simulink model "problem2"  (R2020a)
settings: Solver=VariableStepAuto  StartTime=0.0  StopTime=100  RelTol=1e-3
model workspace (MAT data in the model file):
  b = 350
  k1 = 80000
  k2 = 500000
  m1 = 2500
  m2 = 320
settings Model: OrderedModelArguments=off  Creator=Jake  LastModifiedBy=Jake
settings DataIOCC: ExternalInput=[t,input ]  LoadExternalInput=on

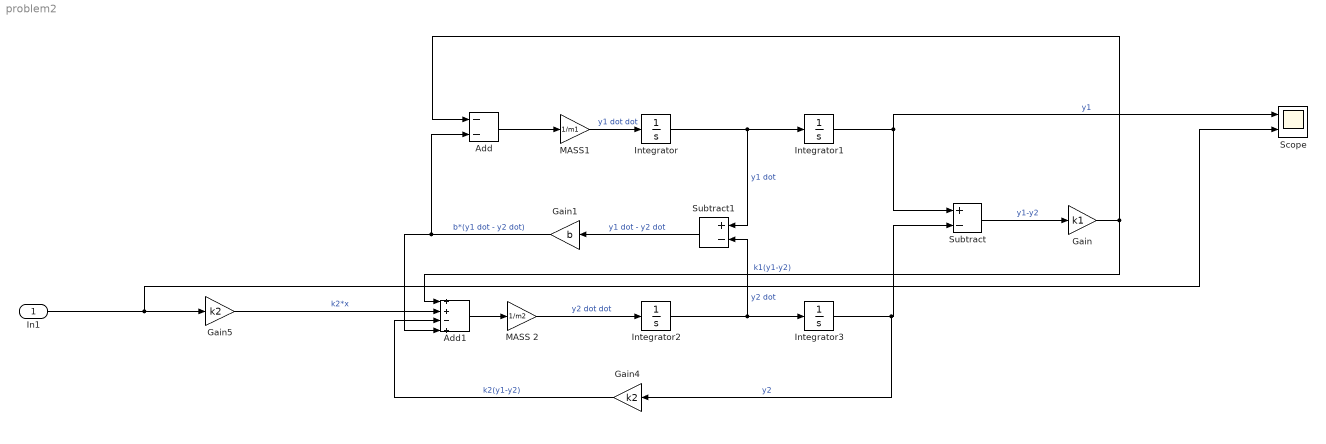
== system problem2 ==
  In1 : Inport
  Add : Sum  Inputs=--
  Add1 : Sum  Inputs=++-+
  Gain : Gain  Gain=k1
  Gain1 : Gain  Gain=b
  Gain4 : Gain  Gain=k2
  Gain5 : Gain  Gain=k2
  Integrator{,1..3} (4 alike) : Integrator
  MASS 2 : Gain  Gain=1/m2
  MASS1 : Gain  Gain=1/m1
  Scope : Scope  NumInputPorts=2
  Subtract : Sum  Inputs=+-
  Subtract1 : Sum  Inputs=+-
  wires:
  Integrator/1 -> Integrator1/1, Subtract1/1  "y1 dot"
  Integrator1/1 -> Scope/1, Subtract/1  "y1"
  Integrator2/1 -> Subtract1/2, Integrator3/1  "y2 dot"
  Integrator3/1 -> Gain4/1, Subtract/2  "y2"
  Subtract/1 -> Gain/1  "y1-y2"
  Subtract1/1 -> Gain1/1  "y1 dot - y2 dot"
  MASS1/1 -> Integrator/1  "y1 dot dot"
  Add/1 -> MASS1/1
  Gain/1 -> Add1/1, Add/1  "k1(y1-y2)"
  Gain1/1 -> Add1/4, Add/2  "b*(y1 dot - y2 dot)"
  MASS 2/1 -> Integrator2/1  "y2 dot dot"
  Add1/1 -> MASS 2/1
  Gain4/1 -> Add1/3  "k2(y1-y2)"
  In1/1 -> Scope/2, Gain5/1
  Gain5/1 -> Add1/2  "k2*x"
